simulink model "Diesel_Genset_Test_System"  (Simulink 8.1)
settings: Solver=ode3  SolverMode=SingleTasking  StartTime=0.0  StopTime=150  FixedStep=Ts  RelTol=1e-3
PostLoadFcn:
  | Ts=50e-6;SIM_HIL=0;
InitFcn:
  | Ts=50e-6;SIM_HIL=0;
undefined symbols (not defined in the file): fdesignblkfcn, gcbh, Gen_900kW_external_control, HIL_GenSet, Left, ph, type, V
libraries: powerlib x31, powerlib_extras x24, rtio_opalrt_common x19, simulink x17, dspsigops x6, breakers_1ph_3ph x6, rtio_generic_modbus x6, cables_lib x5, rteventslib x4, simulink_extras x3, rtlab x2, ssn_lib x2
(part 3 of 3)

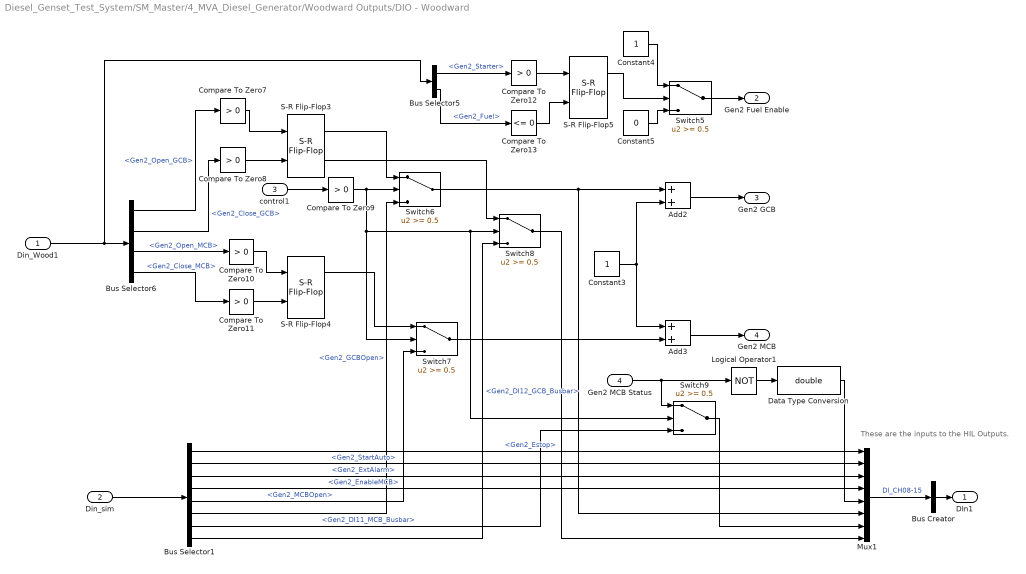
== system Diesel_Genset_Test_System/SM_Master/4_MVA_Diesel_Generator/Woodward Outputs/DIO - Woodward ==
  note: These are the inputs to
      | the HIL Outputs.
  Din_Wood1 : Inport
  Din_sim : Inport  Port=2
  control1 : Inport  Port=3
  Gen2 MCB Status : Inport  Port=4
  Add2 : Sum
  Add3 : Sum
  Bus Creator : BusCreator  Inputs=1
  Bus Selector1 : BusSelector  OutputSignals=16 DOUT GR3.08-11.Gen2_Estop,16 DOUT GR3.08-11.Gen2_StartAuto,16 DOUT GR3.08-11.Gen2_ExtAlarm,16 DOUT GR3.08-11.Gen2_EnableMCB,16 DOUT GR3.12-15.Gen2_MCBOpen,16 DOUT GR3.12-15.Gen2_GCBOpen,16 DOUT GR3.12-15.Gen2_DI11_MCB_Busbar,16 DOUT GR3.12-15.Gen2_DI12_GCB_Busbar
  Bus Selector5 : BusSelector  OutputSignals=DI_CH08-15.Gen2_Starter,DI_CH08-15.Gen2_Fuel
  Bus Selector6 : BusSelector  OutputSignals=DI_CH08-15.Gen2_Open_GCB,DI_CH08-15.Gen2_Close_GCB,DI_CH08-15.Gen2_Open_MCB,DI_CH08-15.Gen2_Close_MCB
  Compare To Zero{7..12} (6 alike) : simulink/Logic and Bit Operations/Compare To Zero  relop=>  OutDataTypeStr=boolean
  Compare To Zero13 : simulink/Logic and Bit Operations/Compare To Zero  relop=<=  OutDataTypeStr=boolean
  Constant3 : Constant
  Constant4 : Constant
  Constant5 : Constant  Value=0
  Data Type Conversion : DataTypeConversion  OutDataTypeStr=double
  Logical Operator1 : Logic  Operator=NOT  AllPortsSameDT=off  OutDataTypeStr=boolean
  Mux1 : Mux  Inputs=8
  S-R Flip-Flop3 : simulink_extras/Flip Flops/S-R Flip-Flop  initial_condition=1
  S-R Flip-Flop4 : simulink_extras/Flip Flops/S-R Flip-Flop  initial_condition=1
  S-R Flip-Flop5 : simulink_extras/Flip Flops/S-R Flip-Flop  initial_condition=0
  Switch5 : Switch  Threshold=0.5
  Switch{6..9} (4 alike) : Switch  Threshold=0.5  OutDataTypeStr=double
      Switch8 settings: LockScale=on
  DIn1 : Outport
  Gen2 Fuel Enable : Outport  Port=2
  Gen2 GCB : Outport  Port=3
  Gen2 MCB : Outport  Port=4
  wires:
  Din_Wood1/1 -> Bus Selector5/1, Bus Selector6/1
  Bus Creator/1 -> DIn1/1
  Mux1/1 -> Bus Creator/1  "DI_CH08-15"
  control1/1 -> Compare To Zero9/1
  S-R Flip-Flop3/1 -> Switch6/1
  Switch6/1 -> Add2/1, Mux1/6
  Bus Selector6/1 -> Compare To Zero7/1  "<Gen2_Open_GCB>"
  Compare To Zero7/1 -> S-R Flip-Flop3/1
  Compare To Zero8/1 -> S-R Flip-Flop3/2
  Bus Selector6/4 -> Compare To Zero11/1  "<Gen2_Close_MCB>"
  Compare To Zero11/1 -> S-R Flip-Flop4/2
  Bus Selector6/3 -> Compare To Zero10/1  "<Gen2_Open_MCB>"
  Compare To Zero10/1 -> S-R Flip-Flop4/1
  S-R Flip-Flop4/1 -> Switch7/1
  Bus Selector6/2 -> Compare To Zero8/1  "<Gen2_Close_GCB>"
  Compare To Zero9/1 -> Switch6/2, Switch7/2, Switch8/2, Switch9/2
  Switch7/1 -> Add3/2
  S-R Flip-Flop3/2 -> Switch8/1
  Add2/1 -> Gen2 GCB/1
  Add3/1 -> Gen2 MCB/1
  Constant3/1 -> Add2/2, Add3/1
  Bus Selector5/1 -> Compare To Zero12/1  "<Gen2_Starter>"
  Bus Selector5/2 -> Compare To Zero13/1  "<Gen2_Fuel>"
  S-R Flip-Flop5/1 -> Switch5/2
  Compare To Zero12/1 -> S-R Flip-Flop5/1
  Constant5/1 -> Switch5/3
  Constant4/1 -> Switch5/1
  Compare To Zero13/1 -> S-R Flip-Flop5/2
  Switch5/1 -> Gen2 Fuel Enable/1
  Bus Selector1/1 -> Mux1/1  "<Gen2_Estop>"
  Bus Selector1/2 -> Mux1/2  "<Gen2_StartAuto>"
  Bus Selector1/3 -> Mux1/3  "<Gen2_ExtAlarm>"
  Bus Selector1/4 -> Mux1/4  "<Gen2_EnableMCB>"
  Bus Selector1/5 -> Switch7/3  "<Gen2_MCBOpen>"
  Bus Selector1/6 -> Switch6/3  "<Gen2_GCBOpen>"
  Din_sim/1 -> Bus Selector1/1
  Bus Selector1/7 -> Switch9/3  "<Gen2_DI11_MCB_Busbar>"
  Switch9/1 -> Mux1/7
  Bus Selector1/8 -> Switch8/3  "<Gen2_DI12_GCB_Busbar>"
  Switch8/1 -> Mux1/8
  Gen2 MCB Status/1 -> Logical Operator1/1, Switch9/1
  Logical Operator1/1 -> Data Type Conversion/1
  Data Type Conversion/1 -> Mux1/5

== system Diesel_Genset_Test_System/SM_Master/4_MVA_Diesel_Generator/Woodward Outputs/DOUT type config ==
  note: The Constants are used to select Digital Output type:
      | - 0: Time-Stamped Digital Output
      | - 1: Pulse-Width Modulated DIgital Output
  DataIn Send : rtio_opalrt_common/DataIn Send  CtrlName='OpCtrl'  FcnNos=11  width=1  portType=double  checkVersion=off  expectedId=0  expectedVersion=0  opComp=>=
      settings: AttributesFormatString=%<CtrlName>
  DataIn Send1 : rtio_opalrt_common/DataIn Send  CtrlName='OpCtrl'  FcnNos=12  width=1  portType=double  checkVersion=off  expectedId=0  expectedVersion=0  opComp=>=
      settings: AttributesFormatString=%<CtrlName>
  Subsection 3 DOUT type : Constant
  Subsection 4 DOUT type : Constant
  Terminator1 : Terminator
  Terminator2 : Terminator
  wires:
  Subsection 3 DOUT type/1 -> DataIn Send/1
  Subsection 4 DOUT type/1 -> DataIn Send1/1
  DataIn Send1/1 -> Terminator1/1
  DataIn Send/1 -> Terminator2/1

== system Diesel_Genset_Test_System/SM_Master/4_MVA_Diesel_Generator/Woodward Outputs/PWM IO - Gr3 ==
  PWMOut : Inport
  Bus Creator : BusCreator  Inputs=2
  Bus Creator1 : BusCreator  Inputs=2
  Bus Creator2 : BusCreator  Inputs=2
  Bus Selector : BusSelector  OutputSignals=FreqPWMOut16-23,DutyPWMOut16-23
  Bus Selector1 : BusSelector  OutputSignals=FreqPWMOut24-31,DutyPWMOut24-31
  Bus Selector2 : BusSelector  OutputSignals=16 PWMOUT GR3.Ch16-23,16 PWMOUT GR3.Ch24-31
  PWM In : rtio_opalrt_common/PWM In  CtrlName='OpCtrl'  portNb=9  FcnNos=Slot 3 Module A Subsection 3  maxCount=8  Count=8  sampleTime=0  numchan=8
      settings: AttributesFormatString=%<CtrlName>
  PWM In1 : rtio_opalrt_common/PWM In  CtrlName='OpCtrl'  portNb=10  FcnNos=Slot 3 Module A Subsection 4  maxCount=8  Count=8  sampleTime=0  numchan=8
      settings: AttributesFormatString=%<CtrlName>
  PWM Out : rtio_opalrt_common/PWM Out  CtrlName='OpCtrl'  portNb=9  FcnNos=Slot 3 Module B Subsection 3  size=64  maxcount=8  count=8  polarity=Active High  symMode=Symmetric  complementary=off  deadTime=0  numchan=8  loadnb=1  initphase=[0 0 0 0 0 0 0 0]
      settings: AttributesFormatString=%<CtrlName>
  PWM Out1 : rtio_opalrt_common/PWM Out  CtrlName='OpCtrl'  portNb=10  FcnNos=Slot 3 Module B Subsection 4  size=64  maxcount=8  count=8  polarity=Active High  symMode=Symmetric  complementary=off  deadTime=0  numchan=8  loadnb=2  initphase=[0 0 0 0 0 0 0 0]
      settings: AttributesFormatString=%<CtrlName>
  Terminator{,1,4..5} (4 alike) : Terminator
  PWMIn : Outport
  wires:
  Bus Selector/1 -> PWM Out/1  "<FreqPWMOut16-23>"
  Bus Selector/2 -> PWM Out/2  "<DutyPWMOut16-23>"
  PWM Out/1 -> Terminator/1
  Bus Selector1/1 -> PWM Out1/1  "<FreqPWMOut24-31>"
  Bus Selector1/2 -> PWM Out1/2  "<DutyPWMOut24-31>"
  PWM Out1/1 -> Terminator1/1
  PWMOut/1 -> Bus Selector2/1
  Bus Selector2/1 -> Bus Selector/1  "<Ch16-23>"
  Bus Creator/1 -> PWMIn/1
  Bus Creator1/1 -> Bus Creator/1  "PWMI_CH16-23"
  Bus Creator2/1 -> Bus Creator/2  "PWMI_CH24-31"
  PWM In1/3 -> Terminator5/1
  PWM In/3 -> Terminator4/1
  PWM In/1 -> Bus Creator1/1  "Freq"
  PWM In/2 -> Bus Creator1/2  "Duty"
  PWM In1/1 -> Bus Creator2/1  "Freq"
  PWM In1/2 -> Bus Creator2/2  "Duty"
  Bus Selector2/2 -> Bus Selector1/1  "<Ch24-31>"

== system Diesel_Genset_Test_System/SM_Master/4_MVA_Diesel_Generator/Woodward Outputs/TSDIO - Gr3 ==
  TSDout : Inport
  Bus Creator : BusCreator  Inputs=16
  Bus Creator1 : BusCreator  Inputs=16
  Bus Creator2 : BusCreator  Inputs=2
  Bus Selector : BusSelector  OutputSignals=16 TSDOUT GR3.states.CH16-23.states 17,16 TSDOUT GR3.times CH16-23.times17,16 TSDOUT GR3.states.CH16-23.states 18,16 TSDOUT GR3.times CH16-23.times18,16 TSDOUT GR3.states.CH16-23.states 19,16 TSDOUT GR3.times CH16-23.times19,16 TSDOUT GR3.states.CH16-23.states 20,16 TSDOUT GR3.times CH16-23.times20,16 TSDOUT GR3.states.CH16-23.states 21,16 TSDOUT GR3.times CH16-23.times21,16 TSDOUT GR3.states.CH16-23.states 22,16 TSDOUT GR3.times CH16-23.times22,16 TSDOUT GR3.states.CH16-23.states 23,16 TSDOUT GR3.times CH16-23.times23,16 TSDOUT GR3.states.CH16-23.states 24,16 TSDOUT GR3.times CH16-23.times24
  Bus Selector1 : BusSelector  OutputSignals=16 TSDOUT GR3.states.CH24-31.states 25,16 TSDOUT GR3.times CH24-31.times25,16 TSDOUT GR3.states.CH24-31.states 26,16 TSDOUT GR3.times CH24-31.times26,16 TSDOUT GR3.states.CH24-31.states 27,16 TSDOUT GR3.times CH24-31.times27,16 TSDOUT GR3.states.CH24-31.states 28,16 TSDOUT GR3.times CH24-31.times28,16 TSDOUT GR3.states.CH24-31.states 29,16 TSDOUT GR3.times CH24-31.times29,16 TSDOUT GR3.states.CH24-31.states 30,16 TSDOUT GR3.times CH24-31.times30,16 TSDOUT GR3.states.CH24-31.states 31,16 TSDOUT GR3.times CH24-31.times31,16 TSDOUT GR3.states.CH24-31.states 32,16 TSDOUT GR3.times CH24-31.times32
  EventDetector : rtio_opalrt_common/EventDetector  CtrlName='OpCtrl'  portNb=7  FcnNos=Slot 3 Module A Subsection 3  size=32  maxcount=8  nbChannels=8  width=4  timeUnit=Time ratio  sampleTime=0  numwidth=4
      settings: AttributesFormatString=%<CtrlName>
  EventDetector1 : rtio_opalrt_common/EventDetector  CtrlName='OpCtrl'  portNb=8  FcnNos=Slot 3 Module A Subsection 4  size=32  maxcount=8  nbChannels=8  width=4  timeUnit=Time ratio  sampleTime=0  numwidth=4
      settings: AttributesFormatString=%<CtrlName>
  EventGenerator : rtio_opalrt_common/EventGenerator  CtrlName='OpCtrl'  portNb=7  FcnNos=Slot 3 Module B Subsection 3  size=32  count=8  nbChannels=8  width=4  timeUnit=Time ratio  numwidth=4
      settings: AttributesFormatString=%<CtrlName>
  EventGenerator1 : rtio_opalrt_common/EventGenerator  CtrlName='OpCtrl'  portNb=8  FcnNos=Slot 3 Module B Subsection 4  size=32  count=8  nbChannels=8  width=4  timeUnit=Time ratio  numwidth=4
      settings: AttributesFormatString=%<CtrlName>
  Terminator{,1..3} (4 alike) : Terminator
  TSDin : Outport
  wires:
  TSDout/1 -> Bus Selector/1, Bus Selector1/1
  Bus Selector/16 -> EventGenerator/16  "<times24>"
  Bus Selector/15 -> EventGenerator/15  "<states 24>"
  Bus Selector/14 -> EventGenerator/14  "<times23>"
  Bus Selector/13 -> EventGenerator/13  "<states 23>"
  Bus Selector/12 -> EventGenerator/12  "<times22>"
  Bus Selector/11 -> EventGenerator/11  "<states 22>"
  Bus Selector/10 -> EventGenerator/10  "<times21>"
  Bus Selector/9 -> EventGenerator/9  "<states 21>"
  Bus Selector/8 -> EventGenerator/8  "<times20>"
  Bus Selector/7 -> EventGenerator/7  "<states 20>"
  Bus Selector/6 -> EventGenerator/6  "<times19>"
  Bus Selector/5 -> EventGenerator/5  "<states 19>"
  Bus Selector/4 -> EventGenerator/4  "<times18>"
  Bus Selector/3 -> EventGenerator/3  "<states 18>"
  Bus Selector/2 -> EventGenerator/2  "<times17>"
  Bus Selector/1 -> EventGenerator/1  "<states 17>"
  EventGenerator/1 -> Terminator/1
  EventDetector/16 -> Bus Creator/16  "times8"
  EventDetector/15 -> Bus Creator/15  "states8"
  EventDetector/14 -> Bus Creator/14  "times7"
  EventDetector/13 -> Bus Creator/13  "states7"
  EventDetector/12 -> Bus Creator/12  "times6"
  EventDetector/11 -> Bus Creator/11  "states6"
  EventDetector/10 -> Bus Creator/10  "times5"
  EventDetector/9 -> Bus Creator/9  "states5"
  EventDetector/8 -> Bus Creator/8  "times4"
  EventDetector/7 -> Bus Creator/7  "states4"
  EventDetector/6 -> Bus Creator/6  "times3"
  EventDetector/5 -> Bus Creator/5  "states3"
  EventDetector/4 -> Bus Creator/4  "times2"
  EventDetector/3 -> Bus Creator/3  "states2"
  EventDetector/2 -> Bus Creator/2  "times1"
  EventDetector/1 -> Bus Creator/1  "states1"
  EventDetector/17 -> Terminator1/1
  EventGenerator1/1 -> Terminator2/1
  Bus Selector1/1 -> EventGenerator1/1  "<states 25>"
  Bus Selector1/2 -> EventGenerator1/2  "<times25>"
  Bus Selector1/3 -> EventGenerator1/3  "<states 26>"
  Bus Selector1/4 -> EventGenerator1/4  "<times26>"
  Bus Selector1/5 -> EventGenerator1/5  "<states 27>"
  Bus Selector1/6 -> EventGenerator1/6  "<times27>"
  Bus Selector1/7 -> EventGenerator1/7  "<states 28>"
  Bus Selector1/8 -> EventGenerator1/8  "<times28>"
  Bus Selector1/9 -> EventGenerator1/9  "<states 29>"
  Bus Selector1/10 -> EventGenerator1/10  "<times29>"
  Bus Selector1/11 -> EventGenerator1/11  "<states 30>"
  Bus Selector1/12 -> EventGenerator1/12  "<times30>"
  Bus Selector1/13 -> EventGenerator1/13  "<states 31>"
  Bus Selector1/14 -> EventGenerator1/14  "<times31>"
  Bus Selector1/15 -> EventGenerator1/15  "<states 32>"
  Bus Selector1/16 -> EventGenerator1/16  "<times32>"
  Bus Creator1/1 -> Bus Creator2/2  "CH24-31"
  EventDetector1/16 -> Bus Creator1/16  "times6"
  EventDetector1/15 -> Bus Creator1/15  "states6"
  EventDetector1/14 -> Bus Creator1/14  "times5"
  EventDetector1/13 -> Bus Creator1/13  "states5"
  EventDetector1/12 -> Bus Creator1/12  "times4"
  EventDetector1/11 -> Bus Creator1/11  "states4"
  EventDetector1/10 -> Bus Creator1/10  "times3"
  EventDetector1/9 -> Bus Creator1/9  "states3"
  EventDetector1/8 -> Bus Creator1/8  "times2"
  EventDetector1/7 -> Bus Creator1/7  "states2"
  EventDetector1/6 -> Bus Creator1/6  "times1"
  EventDetector1/5 -> Bus Creator1/5  "states1"
  EventDetector1/4 -> Bus Creator1/4  "times2"
  EventDetector1/3 -> Bus Creator1/3  "states2"
  EventDetector1/2 -> Bus Creator1/2  "times1"
  EventDetector1/1 -> Bus Creator1/1  "states1"
  EventDetector1/17 -> Terminator3/1  "states7"
  Bus Creator/1 -> Bus Creator2/1  "CH16-23"
  Bus Creator2/1 -> TSDin/1  "TSDIN"

== system Diesel_Genset_Test_System/SM_Master/4_MVA_Diesel_Generator/Woodward Outputs/Woodward Primary Inputs ==
  Bias-ctrl : Inport
  Bus Creator1 : BusCreator
  Constant10 : Constant  Value=1.00
  Constant11 : Constant  Value=1.00
  Constant6 : Constant  Value=0
  Constant7 : Constant  Value=20
  Constant8 : Constant  Value=0
  Constant9 : Constant  Value=0
  Demux1 : Demux  Outputs=16
  Divide2 : Product  Inputs=*/
  Divide3 : Product  Inputs=*/
  GR1 B AIN (CH00-15)1 : Subsystem
  Lowpass Filter2 : Subsystem  DialogController=fdesignblkfcn  DialogControllerArgs=DataTag2  InitFcn=fdesignblkfcn(gcbh, {'InitFcn'});  mask(Lowpass Filter){}
      mask help: Design a lowpass filter
      settings: CopyFcn=fdesignblkfcn(gcbh, {'CopyFcn'});
      mask Help: helpview(mapfilelocation('dsp'), 'dsplowpassfilter');
      mask Display: disp('Lowpass')
  Lowpass Filter3 : Subsystem  DialogController=fdesignblkfcn  DialogControllerArgs=DataTag4  InitFcn=fdesignblkfcn(gcbh, {'InitFcn'});  mask(Lowpass Filter){}
      mask help: Design a lowpass filter
      settings: CopyFcn=fdesignblkfcn(gcbh, {'CopyFcn'});
      mask Help: helpview(mapfilelocation('dsp'), 'dsplowpassfilter');
      mask Display: disp('Lowpass')
  Sum2 : Sum  Inputs=|+-
  Sum3 : Sum  Inputs=|+-
  Switch2 : Switch  Threshold=0.5
  Switch3 : Switch  Threshold=0.5
  Gen2 Gov and AVR : Outport
  wires:
  GR1 B AIN (CH00-15)1/1(Out1) -> [AINs_Gr1], Demux1/1
  Bias-ctrl/1 -> Switch2/2, Switch3/2
  Demux1/3 -> Divide2/1
  Demux1/4 -> Divide3/1
  Constant7/1 -> Divide3/2, Divide2/2
  Divide2/1 -> Sum2/1
  Divide3/1 -> Sum3/1
  Constant8/1 -> Sum2/2
  Constant9/1 -> Sum3/2
  Sum2/1 -> Lowpass Filter2/1(In)
  Switch2/1 -> Bus Creator1/3  "Gen2 GOV"
  Switch3/1 -> Bus Creator1/4  "Gen2 AVR"
  Sum3/1 -> Lowpass Filter3/1(In)
  Constant6/1 -> Switch2/3, Switch3/3
  Lowpass Filter2/1(Out) -> Switch2/1
  Lowpass Filter3/1(Out) -> Switch3/1
  Constant11/1 -> Bus Creator1/2  "Gen2 Ref AVR"
  Constant10/1 -> Bus Creator1/1  "Gen2 Ref GOV"
  Bus Creator1/1 -> Gen2 Gov and AVR/1

== system Diesel_Genset_Test_System/SM_Master/MODBUS1/SEL_787_Relay/PQ_Calculator ==
  Vabc : Inport
  Iabc : Inport  Port=2
  3-phase  Instantaneous  Active & Reactive Power : powerlib_extras/Measurements/3-phase  Instantaneous  Active & Reactive Power
  Demux : Demux  Outputs=2
  Discrete  Mean value2 : powerlib_extras/Discrete Measurements/Discrete  Mean value  Freq=60  Vinit=0  Ts=Ts
  P : Outport
  Q : Outport  Port=2
  wires:
  3-phase  Instantaneous  Active & Reactive Power/1 -> Discrete  Mean value2/1
  Discrete  Mean value2/1 -> Demux/1
  Vabc/1 -> 3-phase  Instantaneous  Active & Reactive Power/1
  Iabc/1 -> 3-phase  Instantaneous  Active & Reactive Power/2
  Demux/1 -> P/1  "P"
  Demux/2 -> Q/1  "Q"

== system Diesel_Genset_Test_System/SM_Master/MODBUS1/SEL_787_Relay/RMS_Calculator ==
  Signal : Inport
  Discrete  Mean value6 : powerlib_extras/Discrete Measurements/Discrete  Mean value  Freq=60  Vinit=0  Ts=Ts
  Product3 : Product  RndMeth=Zero
  Signed Sqrt : Sqrt  SaturateOnIntegerOverflow=on
  RMS_Signal : Outport
  wires:
  Signal/1 -> Product3/1, Product3/2
  Product3/1 -> Discrete  Mean value6/1
  Discrete  Mean value6/1 -> Signed Sqrt/1
  Signed Sqrt/1 -> RMS_Signal/1

== system Diesel_Genset_Test_System/SM_Master/MODBUS1/SEL_787_Relay/RMS_Calculator1 ==
  Signal : Inport
  Discrete  Mean value6 : powerlib_extras/Discrete Measurements/Discrete  Mean value  Freq=60  Vinit=0  Ts=Ts
  Product3 : Product  RndMeth=Zero
  Signed Sqrt : Sqrt  SaturateOnIntegerOverflow=on
  RMS_Signal : Outport
  wires:
  Signal/1 -> Product3/1, Product3/2
  Product3/1 -> Discrete  Mean value6/1
  Discrete  Mean value6/1 -> Signed Sqrt/1
  Signed Sqrt/1 -> RMS_Signal/1

== system Diesel_Genset_Test_System/SM_Master/MODBUS1/SEL_787_Relay/pf_Calculator ==
  P : Inport
  Q : Inport  Port=2
  Fcn : Fcn  Expr=u(1) / sqrt(u(1)^2 + u(2)^2)
  Fcn1 : Fcn  Expr=sqrt(u(1)^2 + u(2)^2)
  Mux : Mux  Inputs=2
  Mux1 : Mux  Inputs=2
  Scope : Scope
      settings: YMin=0.8475  YMax=0.875  SaveName=ScopeData2
  pf : Outport
  S : Outport  Port=2
  wires:
  Fcn1/1 -> S/1
  Mux1/1 -> Fcn1/1
  Fcn/1 -> Scope/1, pf/1
  Mux/1 -> Fcn/1
  P/1 -> Mux1/1, Mux/1
  Q/1 -> Mux1/2, Mux/2

== system Diesel_Genset_Test_System/SM_Master/MODBUS2/SEL_787_Relay/PQ_Calculator ==
  Vabc : Inport
  Iabc : Inport  Port=2
  3-phase  Instantaneous  Active & Reactive Power : powerlib_extras/Measurements/3-phase  Instantaneous  Active & Reactive Power
  Demux : Demux  Outputs=2
  Discrete  Mean value2 : powerlib_extras/Discrete Measurements/Discrete  Mean value  Freq=60  Vinit=0  Ts=Ts
  P : Outport
  Q : Outport  Port=2
  wires:
  3-phase  Instantaneous  Active & Reactive Power/1 -> Discrete  Mean value2/1
  Discrete  Mean value2/1 -> Demux/1
  Vabc/1 -> 3-phase  Instantaneous  Active & Reactive Power/1
  Iabc/1 -> 3-phase  Instantaneous  Active & Reactive Power/2
  Demux/1 -> P/1  "P"
  Demux/2 -> Q/1  "Q"

== system Diesel_Genset_Test_System/SM_Master/MODBUS2/SEL_787_Relay/RMS_Calculator ==
  Signal : Inport
  Discrete  Mean value6 : powerlib_extras/Discrete Measurements/Discrete  Mean value  Freq=60  Vinit=0  Ts=Ts
  Product3 : Product  RndMeth=Zero
  Signed Sqrt : Sqrt  SaturateOnIntegerOverflow=on
  RMS_Signal : Outport
  wires:
  Signal/1 -> Product3/1, Product3/2
  Product3/1 -> Discrete  Mean value6/1
  Discrete  Mean value6/1 -> Signed Sqrt/1
  Signed Sqrt/1 -> RMS_Signal/1

== system Diesel_Genset_Test_System/SM_Master/MODBUS2/SEL_787_Relay/RMS_Calculator1 ==
  Signal : Inport
  Discrete  Mean value6 : powerlib_extras/Discrete Measurements/Discrete  Mean value  Freq=60  Vinit=0  Ts=Ts
  Product3 : Product  RndMeth=Zero
  Signed Sqrt : Sqrt  SaturateOnIntegerOverflow=on
  RMS_Signal : Outport
  wires:
  Signal/1 -> Product3/1, Product3/2
  Product3/1 -> Discrete  Mean value6/1
  Discrete  Mean value6/1 -> Signed Sqrt/1
  Signed Sqrt/1 -> RMS_Signal/1

== system Diesel_Genset_Test_System/SM_Master/MODBUS2/SEL_787_Relay/pf_Calculator ==
  P : Inport
  Q : Inport  Port=2
  Fcn : Fcn  Expr=u(1) / sqrt(u(1)^2 + u(2)^2)
  Fcn1 : Fcn  Expr=sqrt(u(1)^2 + u(2)^2)
  Mux : Mux  Inputs=2
  Mux1 : Mux  Inputs=2
  Scope : Scope
      settings: YMin=0.8475  YMax=0.875  SaveName=ScopeData2
  pf : Outport
  S : Outport  Port=2
  wires:
  Fcn1/1 -> S/1
  Mux1/1 -> Fcn1/1
  Fcn/1 -> Scope/1, pf/1
  Mux/1 -> Fcn/1
  P/1 -> Mux1/1, Mux/1
  Q/1 -> Mux1/2, Mux/2

== system Diesel_Genset_Test_System/SM_Master/MODBUS4/SEL_787_Relay/PQ_Calculator ==
  Vabc : Inport
  Iabc : Inport  Port=2
  3-phase  Instantaneous  Active & Reactive Power : powerlib_extras/Measurements/3-phase  Instantaneous  Active & Reactive Power
  Demux : Demux  Outputs=2
  Discrete  Mean value2 : powerlib_extras/Discrete Measurements/Discrete  Mean value  Freq=60  Vinit=0  Ts=Ts
  P : Outport
  Q : Outport  Port=2
  wires:
  3-phase  Instantaneous  Active & Reactive Power/1 -> Discrete  Mean value2/1
  Discrete  Mean value2/1 -> Demux/1
  Vabc/1 -> 3-phase  Instantaneous  Active & Reactive Power/1
  Iabc/1 -> 3-phase  Instantaneous  Active & Reactive Power/2
  Demux/1 -> P/1  "P"
  Demux/2 -> Q/1  "Q"

== system Diesel_Genset_Test_System/SM_Master/MODBUS4/SEL_787_Relay/RMS_Calculator ==
  Signal : Inport
  Discrete  Mean value6 : powerlib_extras/Discrete Measurements/Discrete  Mean value  Freq=60  Vinit=0  Ts=Ts
  Product3 : Product  RndMeth=Zero
  Signed Sqrt : Sqrt  SaturateOnIntegerOverflow=on
  RMS_Signal : Outport
  wires:
  Signal/1 -> Product3/1, Product3/2
  Product3/1 -> Discrete  Mean value6/1
  Discrete  Mean value6/1 -> Signed Sqrt/1
  Signed Sqrt/1 -> RMS_Signal/1

== system Diesel_Genset_Test_System/SM_Master/MODBUS4/SEL_787_Relay/RMS_Calculator1 ==
  Signal : Inport
  Discrete  Mean value6 : powerlib_extras/Discrete Measurements/Discrete  Mean value  Freq=60  Vinit=0  Ts=Ts
  Product3 : Product  RndMeth=Zero
  Signed Sqrt : Sqrt  SaturateOnIntegerOverflow=on
  RMS_Signal : Outport
  wires:
  Signal/1 -> Product3/1, Product3/2
  Product3/1 -> Discrete  Mean value6/1
  Discrete  Mean value6/1 -> Signed Sqrt/1
  Signed Sqrt/1 -> RMS_Signal/1

== system Diesel_Genset_Test_System/SM_Master/MODBUS4/SEL_787_Relay/pf_Calculator ==
  P : Inport
  Q : Inport  Port=2
  Fcn : Fcn  Expr=u(1) / sqrt(u(1)^2 + u(2)^2)
  Fcn1 : Fcn  Expr=sqrt(u(1)^2 + u(2)^2)
  Mux : Mux  Inputs=2
  Mux1 : Mux  Inputs=2
  Scope : Scope
      settings: YMin=0.8475  YMax=0.875  SaveName=ScopeData2
  pf : Outport
  S : Outport  Port=2
  wires:
  Fcn1/1 -> S/1
  Mux1/1 -> Fcn1/1
  Fcn/1 -> Scope/1, pf/1
  Mux/1 -> Fcn/1
  P/1 -> Mux1/1, Mux/1
  Q/1 -> Mux1/2, Mux/2

== system Diesel_Genset_Test_System/SM_Master/MODBUS5/SEL_787_Relay/PQ_Calculator ==
  Vabc : Inport
  Iabc : Inport  Port=2
  3-phase  Instantaneous  Active & Reactive Power : powerlib_extras/Measurements/3-phase  Instantaneous  Active & Reactive Power
  Demux : Demux  Outputs=2
  Discrete  Mean value2 : powerlib_extras/Discrete Measurements/Discrete  Mean value  Freq=60  Vinit=0  Ts=Ts
  P : Outport
  Q : Outport  Port=2
  wires:
  3-phase  Instantaneous  Active & Reactive Power/1 -> Discrete  Mean value2/1
  Discrete  Mean value2/1 -> Demux/1
  Vabc/1 -> 3-phase  Instantaneous  Active & Reactive Power/1
  Iabc/1 -> 3-phase  Instantaneous  Active & Reactive Power/2
  Demux/1 -> P/1  "P"
  Demux/2 -> Q/1  "Q"

== system Diesel_Genset_Test_System/SM_Master/MODBUS5/SEL_787_Relay/RMS_Calculator ==
  Signal : Inport
  Discrete  Mean value6 : powerlib_extras/Discrete Measurements/Discrete  Mean value  Freq=60  Vinit=0  Ts=Ts
  Product3 : Product  RndMeth=Zero
  Signed Sqrt : Sqrt  SaturateOnIntegerOverflow=on
  RMS_Signal : Outport
  wires:
  Signal/1 -> Product3/1, Product3/2
  Product3/1 -> Discrete  Mean value6/1
  Discrete  Mean value6/1 -> Signed Sqrt/1
  Signed Sqrt/1 -> RMS_Signal/1

== system Diesel_Genset_Test_System/SM_Master/MODBUS5/SEL_787_Relay/RMS_Calculator1 ==
  Signal : Inport
  Discrete  Mean value6 : powerlib_extras/Discrete Measurements/Discrete  Mean value  Freq=60  Vinit=0  Ts=Ts
  Product3 : Product  RndMeth=Zero
  Signed Sqrt : Sqrt  SaturateOnIntegerOverflow=on
  RMS_Signal : Outport
  wires:
  Signal/1 -> Product3/1, Product3/2
  Product3/1 -> Discrete  Mean value6/1
  Discrete  Mean value6/1 -> Signed Sqrt/1
  Signed Sqrt/1 -> RMS_Signal/1

== system Diesel_Genset_Test_System/SM_Master/MODBUS5/SEL_787_Relay/pf_Calculator ==
  P : Inport
  Q : Inport  Port=2
  Fcn : Fcn  Expr=u(1) / sqrt(u(1)^2 + u(2)^2)
  Fcn1 : Fcn  Expr=sqrt(u(1)^2 + u(2)^2)
  Mux : Mux  Inputs=2
  Mux1 : Mux  Inputs=2
  Scope : Scope
      settings: YMin=0.8475  YMax=0.875  SaveName=ScopeData2
  pf : Outport
  S : Outport  Port=2
  wires:
  Fcn1/1 -> S/1
  Mux1/1 -> Fcn1/1
  Fcn/1 -> Scope/1, pf/1
  Mux/1 -> Fcn/1
  P/1 -> Mux1/1, Mux/1
  Q/1 -> Mux1/2, Mux/2

== system Diesel_Genset_Test_System/SM_Master/MODBUS6/SEL_787_Relay/PQ_Calculator ==
  Vabc : Inport
  Iabc : Inport  Port=2
  3-phase  Instantaneous  Active & Reactive Power : powerlib_extras/Measurements/3-phase  Instantaneous  Active & Reactive Power
  Demux : Demux  Outputs=2
  Discrete  Mean value2 : powerlib_extras/Discrete Measurements/Discrete  Mean value  Freq=60  Vinit=0  Ts=Ts
  P : Outport
  Q : Outport  Port=2
  wires:
  3-phase  Instantaneous  Active & Reactive Power/1 -> Discrete  Mean value2/1
  Discrete  Mean value2/1 -> Demux/1
  Vabc/1 -> 3-phase  Instantaneous  Active & Reactive Power/1
  Iabc/1 -> 3-phase  Instantaneous  Active & Reactive Power/2
  Demux/1 -> P/1  "P"
  Demux/2 -> Q/1  "Q"

== system Diesel_Genset_Test_System/SM_Master/MODBUS6/SEL_787_Relay/RMS_Calculator ==
  Signal : Inport
  Discrete  Mean value6 : powerlib_extras/Discrete Measurements/Discrete  Mean value  Freq=60  Vinit=0  Ts=Ts
  Product3 : Product  RndMeth=Zero
  Signed Sqrt : Sqrt  SaturateOnIntegerOverflow=on
  RMS_Signal : Outport
  wires:
  Signal/1 -> Product3/1, Product3/2
  Product3/1 -> Discrete  Mean value6/1
  Discrete  Mean value6/1 -> Signed Sqrt/1
  Signed Sqrt/1 -> RMS_Signal/1

== system Diesel_Genset_Test_System/SM_Master/MODBUS6/SEL_787_Relay/RMS_Calculator1 ==
  Signal : Inport
  Discrete  Mean value6 : powerlib_extras/Discrete Measurements/Discrete  Mean value  Freq=60  Vinit=0  Ts=Ts
  Product3 : Product  RndMeth=Zero
  Signed Sqrt : Sqrt  SaturateOnIntegerOverflow=on
  RMS_Signal : Outport
  wires:
  Signal/1 -> Product3/1, Product3/2
  Product3/1 -> Discrete  Mean value6/1
  Discrete  Mean value6/1 -> Signed Sqrt/1
  Signed Sqrt/1 -> RMS_Signal/1

== system Diesel_Genset_Test_System/SM_Master/MODBUS6/SEL_787_Relay/pf_Calculator ==
  P : Inport
  Q : Inport  Port=2
  Fcn : Fcn  Expr=u(1) / sqrt(u(1)^2 + u(2)^2)
  Fcn1 : Fcn  Expr=sqrt(u(1)^2 + u(2)^2)
  Mux : Mux  Inputs=2
  Mux1 : Mux  Inputs=2
  Scope : Scope
      settings: YMin=0.8475  YMax=0.875  SaveName=ScopeData2
  pf : Outport
  S : Outport  Port=2
  wires:
  Fcn1/1 -> S/1
  Mux1/1 -> Fcn1/1
  Fcn/1 -> Scope/1, pf/1
  Mux/1 -> Fcn/1
  P/1 -> Mux1/1, Mux/1
  Q/1 -> Mux1/2, Mux/2

== system Diesel_Genset_Test_System/SM_Master/MODBUS8/SEL_787_Relay/PQ_Calculator ==
  Vabc : Inport
  Iabc : Inport  Port=2
  3-phase  Instantaneous  Active & Reactive Power : powerlib_extras/Measurements/3-phase  Instantaneous  Active & Reactive Power
  Demux : Demux  Outputs=2
  Discrete  Mean value2 : powerlib_extras/Discrete Measurements/Discrete  Mean value  Freq=60  Vinit=0  Ts=Ts
  P : Outport
  Q : Outport  Port=2
  wires:
  3-phase  Instantaneous  Active & Reactive Power/1 -> Discrete  Mean value2/1
  Discrete  Mean value2/1 -> Demux/1
  Vabc/1 -> 3-phase  Instantaneous  Active & Reactive Power/1
  Iabc/1 -> 3-phase  Instantaneous  Active & Reactive Power/2
  Demux/1 -> P/1  "P"
  Demux/2 -> Q/1  "Q"

== system Diesel_Genset_Test_System/SM_Master/MODBUS8/SEL_787_Relay/RMS_Calculator ==
  Signal : Inport
  Discrete  Mean value6 : powerlib_extras/Discrete Measurements/Discrete  Mean value  Freq=60  Vinit=0  Ts=Ts
  Product3 : Product  RndMeth=Zero
  Signed Sqrt : Sqrt  SaturateOnIntegerOverflow=on
  RMS_Signal : Outport
  wires:
  Signal/1 -> Product3/1, Product3/2
  Product3/1 -> Discrete  Mean value6/1
  Discrete  Mean value6/1 -> Signed Sqrt/1
  Signed Sqrt/1 -> RMS_Signal/1

== system Diesel_Genset_Test_System/SM_Master/MODBUS8/SEL_787_Relay/RMS_Calculator1 ==
  Signal : Inport
  Discrete  Mean value6 : powerlib_extras/Discrete Measurements/Discrete  Mean value  Freq=60  Vinit=0  Ts=Ts
  Product3 : Product  RndMeth=Zero
  Signed Sqrt : Sqrt  SaturateOnIntegerOverflow=on
  RMS_Signal : Outport
  wires:
  Signal/1 -> Product3/1, Product3/2
  Product3/1 -> Discrete  Mean value6/1
  Discrete  Mean value6/1 -> Signed Sqrt/1
  Signed Sqrt/1 -> RMS_Signal/1

== system Diesel_Genset_Test_System/SM_Master/MODBUS8/SEL_787_Relay/pf_Calculator ==
  P : Inport
  Q : Inport  Port=2
  Fcn : Fcn  Expr=u(1) / sqrt(u(1)^2 + u(2)^2)
  Fcn1 : Fcn  Expr=sqrt(u(1)^2 + u(2)^2)
  Mux : Mux  Inputs=2
  Mux1 : Mux  Inputs=2
  Scope : Scope
      settings: YMin=0.8475  YMax=0.875  SaveName=ScopeData2
  pf : Outport
  S : Outport  Port=2
  wires:
  Fcn1/1 -> S/1
  Mux1/1 -> Fcn1/1
  Fcn/1 -> Scope/1, pf/1
  Mux/1 -> Fcn/1
  P/1 -> Mux1/1, Mux/1
  Q/1 -> Mux1/2, Mux/2

== system Diesel_Genset_Test_System/SC_Console/Woodward/16TSDIn/16 TSDOut GR3/Dout state ctrl/Dout_CH16_CH23 ==
  Bus Creator1 : BusCreator  Inputs=8
  Dout_CH{16..23} (8 alike) : Constant  Value=[1 0 1 0]
  Manual Switch{17..24} (8 alike) : ManualSwitch
  Zero_Dout_CH{16..23} (8 alike) : Constant  Value=[0 0 0 0]
  Dout_CH8_CH15 : Outport
  wires:
  Manual Switch24/1 -> Bus Creator1/8  "states 24"
  Manual Switch23/1 -> Bus Creator1/7  "states 23"
  Manual Switch22/1 -> Bus Creator1/6  "states 22"
  Manual Switch21/1 -> Bus Creator1/5  "states 21"
  Manual Switch20/1 -> Bus Creator1/4  "states 20"
  Manual Switch19/1 -> Bus Creator1/3  "states 19"
  Manual Switch18/1 -> Bus Creator1/2  "states 18"
  Manual Switch17/1 -> Bus Creator1/1  "states 17"
  Zero_Dout_CH23/1 -> Manual Switch24/2
  Dout_CH23/1 -> Manual Switch24/1
  Zero_Dout_CH22/1 -> Manual Switch23/2
  Dout_CH22/1 -> Manual Switch23/1
  Zero_Dout_CH21/1 -> Manual Switch22/2
  Dout_CH21/1 -> Manual Switch22/1
  Zero_Dout_CH20/1 -> Manual Switch21/2
  Dout_CH20/1 -> Manual Switch21/1
  Zero_Dout_CH19/1 -> Manual Switch20/2
  Dout_CH19/1 -> Manual Switch20/1
  Zero_Dout_CH18/1 -> Manual Switch19/2
  Dout_CH18/1 -> Manual Switch19/1
  Zero_Dout_CH17/1 -> Manual Switch18/2
  Dout_CH17/1 -> Manual Switch18/1
  Zero_Dout_CH16/1 -> Manual Switch17/2
  Dout_CH16/1 -> Manual Switch17/1
  Bus Creator1/1 -> Dout_CH8_CH15/1

== system Diesel_Genset_Test_System/SC_Console/Woodward/16TSDIn/16 TSDOut GR3/Dout state ctrl/Dout_CH24_CH31 ==
  Bus Creator : BusCreator  Inputs=8
  Dout_CH{24..31} (8 alike) : Constant  Value=[1 0 1 0]
  Manual Switch{25..32} (8 alike) : ManualSwitch
  Zero_Dout_CH{24..31} (8 alike) : Constant  Value=[0 0 0 0]
  Dout_CH8_CH15 : Outport
  wires:
  Bus Creator/1 -> Dout_CH8_CH15/1
  Dout_CH24/1 -> Manual Switch25/1
  Zero_Dout_CH24/1 -> Manual Switch25/2
  Dout_CH25/1 -> Manual Switch26/1
  Zero_Dout_CH25/1 -> Manual Switch26/2
  Dout_CH26/1 -> Manual Switch27/1
  Zero_Dout_CH26/1 -> Manual Switch27/2
  Dout_CH27/1 -> Manual Switch28/1
  Zero_Dout_CH27/1 -> Manual Switch28/2
  Dout_CH28/1 -> Manual Switch29/1
  Zero_Dout_CH28/1 -> Manual Switch29/2
  Dout_CH29/1 -> Manual Switch30/1
  Zero_Dout_CH29/1 -> Manual Switch30/2
  Dout_CH30/1 -> Manual Switch31/1
  Zero_Dout_CH30/1 -> Manual Switch31/2
  Dout_CH31/1 -> Manual Switch32/1
  Zero_Dout_CH31/1 -> Manual Switch32/2
  Manual Switch25/1 -> Bus Creator/1  "states 25"
  Manual Switch26/1 -> Bus Creator/2  "states 26"
  Manual Switch27/1 -> Bus Creator/3  "states 27"
  Manual Switch28/1 -> Bus Creator/4  "states 28"
  Manual Switch29/1 -> Bus Creator/5  "states 29"
  Manual Switch30/1 -> Bus Creator/6  "states 30"
  Manual Switch31/1 -> Bus Creator/7  "states 31"
  Manual Switch32/1 -> Bus Creator/8  "states 32"

== system Diesel_Genset_Test_System/SM_Master/4_MVA_Diesel_Generator/Woodward Outputs/DIO - Gr3/Conditioning1 ==
  In1 : Inport
  Bus Creator : BusCreator  Inputs=8
  Demux : Demux  Outputs=8
  Out1 : Outport
  wires:
  In1/1 -> Demux/1
  Bus Creator/1 -> Out1/1  "DI_CH08-15"
  Demux/8 -> Bus Creator/8  "Gen2_Alarm_CF"
  Demux/7 -> Bus Creator/7  "Gen2_Alarm_AB"
  Demux/6 -> Bus Creator/6  "Gen2_Open_MCB"
  Demux/5 -> Bus Creator/5  "Gen2_Close_MCB"
  Demux/4 -> Bus Creator/4  "Gen2_Open_GCB"
  Demux/3 -> Bus Creator/3  "Gen2_Close_GCB"
  Demux/2 -> Bus Creator/2  "Gen2_Fuel"
  Demux/1 -> Bus Creator/1  "Gen2_Starter"

== system Diesel_Genset_Test_System/SM_Master/4_MVA_Diesel_Generator/Woodward Outputs/Woodward Primary Inputs/GR1 B AIN (CH00-15)1 ==
  AnalogIn : rtio_opalrt_common/AnalogIn  CtrlName='OpCtrl'  portNb=1  FcnNos=Slot 1 Module B Subsection 1  size=16  maxcount=8  count=8  numchan=8  sampleTime=0
      settings: AttributesFormatString=%<CtrlName>
  AnalogIn1 : rtio_opalrt_common/AnalogIn  CtrlName='OpCtrl'  portNb=2  FcnNos=Slot 1 Module B Subsection 2  size=16  maxcount=8  count=8  numchan=8  sampleTime=0
      settings: AttributesFormatString=%<CtrlName>
  Mux6 : Mux  Inputs=2
  Terminator2 : Terminator
  Terminator3 : Terminator
  Out1 : Outport
  wires:
  AnalogIn/1 -> Mux6/1
  AnalogIn1/1 -> Mux6/2
  AnalogIn/2 -> Terminator2/1
  AnalogIn1/2 -> Terminator3/1
  Mux6/1 -> Out1/1

== system Diesel_Genset_Test_System/SM_Master/4_MVA_Diesel_Generator/Woodward Outputs/Woodward Primary Inputs/Lowpass Filter2 ==
  In : Inport
  Generated Filter Block : DiscreteFir  Tag=BlockMethodSubSystem  Coefficients=[0.0069552863617617106 0.014587901014631248 -0.0057896483056441538 -0.056861876528372622 -0.059476680260783142 0.076118200884714562 0.29579154768342669 0.40638624201187618 0.29579154768342669 0.076118200884714562 -0.059476680260783142 -0.056861876528372622 -0.0057896483056441538 0.014587901014631248 0.0069552863617617106]  InputProcessing=Columns as channels (frame based)
  Out : Outport
  wires:
  In/1 -> Generated Filter Block/1
  Generated Filter Block/1 -> Out/1

== system Diesel_Genset_Test_System/SM_Master/4_MVA_Diesel_Generator/Woodward Outputs/Woodward Primary Inputs/Lowpass Filter3 ==
  In : Inport
  Generated Filter Block : DiscreteFir  Tag=BlockMethodSubSystem  Coefficients=[0.0069552863617617106 0.014587901014631248 -0.0057896483056441538 -0.056861876528372622 -0.059476680260783142 0.076118200884714562 0.29579154768342669 0.40638624201187618 0.29579154768342669 0.076118200884714562 -0.059476680260783142 -0.056861876528372622 -0.0057896483056441538 0.014587901014631248 0.0069552863617617106]  InputProcessing=Columns as channels (frame based)
  Out : Outport
  wires:
  In/1 -> Generated Filter Block/1
  Generated Filter Block/1 -> Out/1
